simulink model "chap2_5sim"  (R2016b)
settings: Solver=ode45  StartTime=0.0  StopTime=RunTime  FixedStep=0.01  RelTol=1e-3  EnableMultiTasking=on
settings Model: Creator=Masoud  LastModifiedBy=IT
settings DataIOCC: LimitDataPoints=on  SaveFormat=Array
settings OptimizationCC: LifeSpan=inf
settings DebuggingCC: AlgebraicLoopMsg=none  ArtificialAlgebraicLoopMsg=none  InheritedTsInSrcMsg=none  SFUnexpectedBacktrackingDiag=warning  SFNoUnconditionalDefaultTransitionDiag=warning  SFExecutionAtInitializationDiag=none
settings HardwareCC: ProdBitPerPointer=32  ProdBitPerSizeT=32  ProdBitPerPtrDiffT=32  ProdLargestAtomicFloat=None  ProdIntDivRoundTo=Undefined  ProdEndianess=Unspecified  ProdWordSize=32  ProdHWDeviceType=32-bit Generic
settings ModelReferenceCC: PropagateSignalLabelsOutOfModel=off
settings GRTTargetCC: TargetLangStandard=C89/C90 (ANSI)  GeneratePreprocessorConditionals=Disable all
settings ConfigComp: CovMetricSettings=dw  CovHtmlReporting=on  CovSaveCumulativeToWorkspaceVar=on  CovSaveSingleToWorkspaceVar=on  CovExternalEMLEnable=off

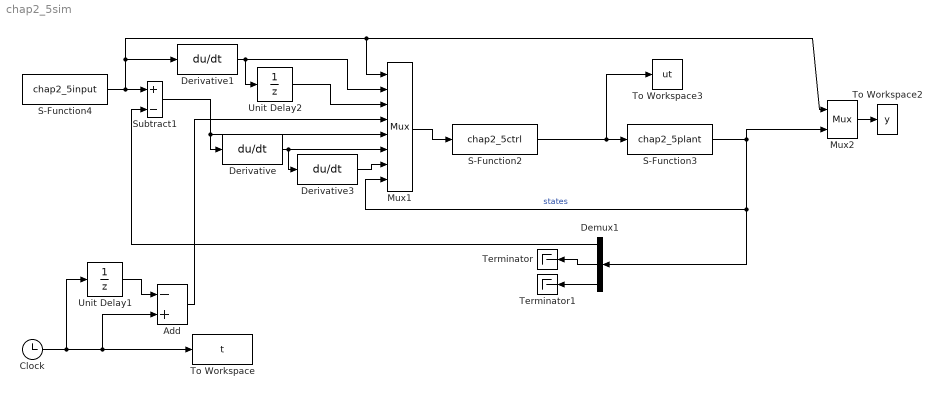
== system chap2_5sim ==
  Add : Sum  Inputs=-+
  Clock : Clock
  Demux1 : Demux  Outputs=3
  Derivative : Derivative
  Derivative1 : Derivative
  Derivative3 : Derivative
  Mux1 : Mux  Inputs=8
  Mux2 : Mux  Inputs=2
  S-Function2 : S-Function  FunctionName=chap2_5ctrl  SFunctionModules='chap2_5ctrl'  SFunctionDeploymentMode=off  EnableBusSupport=off
  S-Function3 : S-Function  FunctionName=chap2_5plant  SFunctionModules='chap2_5plant'  SFunctionDeploymentMode=off  EnableBusSupport=off
  S-Function4 : S-Function  FunctionName=chap2_5input  SFunctionModules='chap2_5input'  SFunctionDeploymentMode=off  EnableBusSupport=off
  Subtract1 : Sum  Inputs=+-
  Terminator : Terminator
  Terminator1 : Terminator
  To Workspace : ToWorkspace  VariableName=t  SampleTime=-1
  To Workspace2 : ToWorkspace  VariableName=y  SampleTime=-1
  To Workspace3 : ToWorkspace  VariableName=ut  SampleTime=-1
  Unit Delay1 : UnitDelay  SampleTime=-1
  Unit Delay2 : UnitDelay  SampleTime=-1
  wires:
  Mux1/1 -> S-Function2/1
  Mux2/1 -> To Workspace2/1
  S-Function3/1 -> Mux2/2, Mux1/8, Demux1/1  "states"
  Demux1/2 -> Terminator/1
  Demux1/3 -> Terminator1/1
  S-Function2/1 -> To Workspace3/1, S-Function3/1
  Demux1/1 -> Subtract1/2
  S-Function4/1 -> Mux1/1, Mux2/1, Derivative1/1, Subtract1/1
  Subtract1/1 -> Mux1/5, Derivative/1
  Derivative/1 -> Mux1/6, Derivative3/1
  Derivative1/1 -> Unit Delay2/1, Mux1/2
  Unit Delay2/1 -> Mux1/3
  Derivative3/1 -> Mux1/7
  Clock/1 -> To Workspace/1, Add/2, Unit Delay1/1
  Add/1 -> Mux1/4
  Unit Delay1/1 -> Add/1
